simulink model "PV_Battery_MPC"  (R2025a)
settings: Solver=ode4  StartTime=0.0  StopTime=ScenarioStopTime  FixedStep=1e-5  RelTol=1e-3
undefined symbols (not defined in the file): ARIMA_Phi_G, ARIMA_Phi_R, ARIMA_Phi_T, BAT_OCV_TABLE, BAT_SOC_BP, ControllerSelect, DC_PI_Ki, DC_PI_Kp, MPC_OV_weights_curtail, MPC_OV_weights_normal, MPPT_P_deadband, MPPT_P_init, MPPT_V_init, MPPT_V_max, MPPT_V_min, MPPT_V_step, OperatingPointInfo, PV_G_BP, PV_I_TABLE, PV_PI_Ki, PV_PI_Kp, PV_T_BP, PV_V_BP, PVBATT_P, u0, w0, x0
libraries: mpclib x1
settings Model: Creator=Limingyu  LastModifiedBy=Limingyu
settings DataIOCC: SaveOutput=off  SignalLogging=off

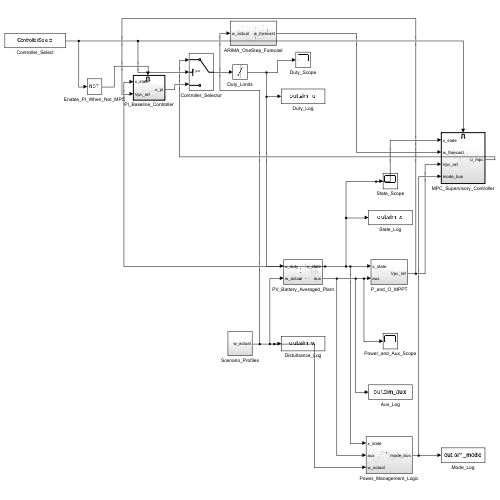
[thumbnail: Simulink's stored preview of the top-level diagram]
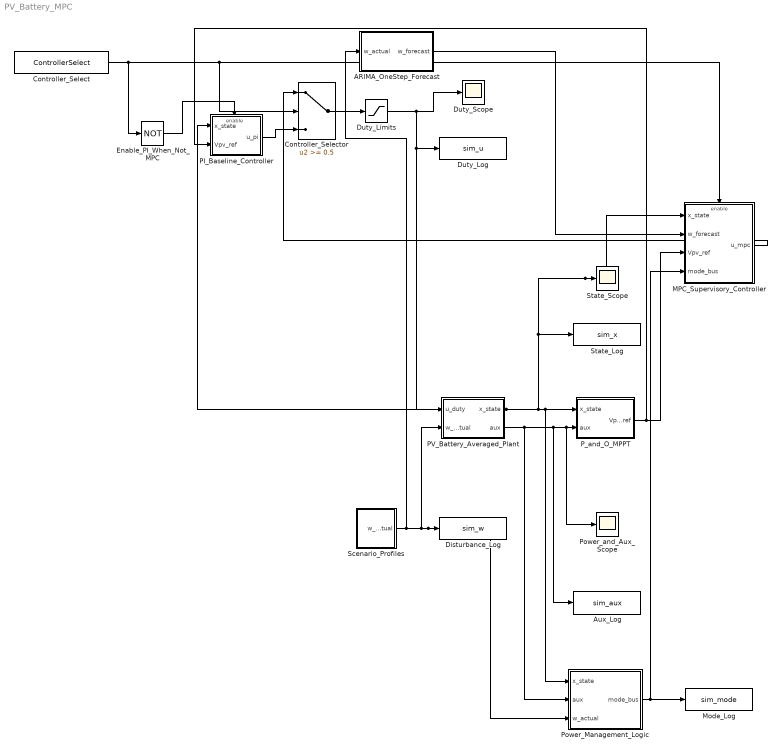
== system PV_Battery_MPC ==
  ARIMA_OneStep_Forecast : Subsystem
  Aux_Log : ToWorkspace  VariableName=sim_aux  SaveFormat=Structure With Time
      settings: Decimation=100
  Controller_Select : Constant  Value=ControllerSelect
  Controller_Selector : Switch  Threshold=0.5
  Disturbance_Log : ToWorkspace  VariableName=sim_w  SaveFormat=Structure With Time
      settings: Decimation=100
  Duty_Limits : Saturate  UpperLimit=0.95  LowerLimit=0.02
  Duty_Log : ToWorkspace  VariableName=sim_u  SaveFormat=Structure With Time
      settings: Decimation=100
  Duty_Scope : Scope
  Enable_PI_When_Not_MPC : Logic  Operator=NOT  Inputs=1  AllPortsSameDT=off  OutDataTypeStr=boolean
  MPC_Supervisory_Controller : Subsystem
  Mode_Log : ToWorkspace  VariableName=sim_mode  SaveFormat=Structure With Time
      settings: Decimation=100
  PI_Baseline_Controller : Subsystem
  PV_Battery_Averaged_Plant : Subsystem
  P_and_O_MPPT : Subsystem
  Power_Management_Logic : Subsystem
  Power_and_Aux_Scope : Scope
  Scenario_Profiles : Subsystem
  State_Log : ToWorkspace  VariableName=sim_x  SaveFormat=Structure With Time
      settings: Decimation=100
  State_Scope : Scope
  wires:
  Duty_Limits/1 -> PV_Battery_Averaged_Plant/1(u_duty), Duty_Log/1, Duty_Scope/1
  Controller_Selector/1 -> Duty_Limits/1
  PI_Baseline_Controller/1(u_pi) -> Controller_Selector/3
  Controller_Select/1 -> Controller_Selector/2, MPC_Supervisory_Controller/Enable, Enable_PI_When_Not_MPC/1
  MPC_Supervisory_Controller/1(u_mpc) -> Controller_Selector/1
  Power_Management_Logic/1(mode_bus) -> MPC_Supervisory_Controller/4(mode_bus), Mode_Log/1
  P_and_O_MPPT/1(Vpv_ref) -> PI_Baseline_Controller/2(Vpv_ref), MPC_Supervisory_Controller/3(Vpv_ref)
  ARIMA_OneStep_Forecast/1(w_forecast) -> MPC_Supervisory_Controller/2(w_forecast)
  PV_Battery_Averaged_Plant/2(aux) -> Aux_Log/1, Power_and_Aux_Scope/1, P_and_O_MPPT/2(aux), Power_Management_Logic/2(aux)
  PV_Battery_Averaged_Plant/1(x_state) -> Power_Management_Logic/1(x_state), P_and_O_MPPT/1(x_state), State_Scope/1, MPC_Supervisory_Controller/1(x_state), State_Log/1, PI_Baseline_Controller/1(x_state)
  Scenario_Profiles/1(w_actual) -> PV_Battery_Averaged_Plant/2(w_actual), Disturbance_Log/1, Power_Management_Logic/3(w_actual), ARIMA_OneStep_Forecast/1(w_actual)
  Enable_PI_When_Not_MPC/1 -> PI_Baseline_Controller/Enable

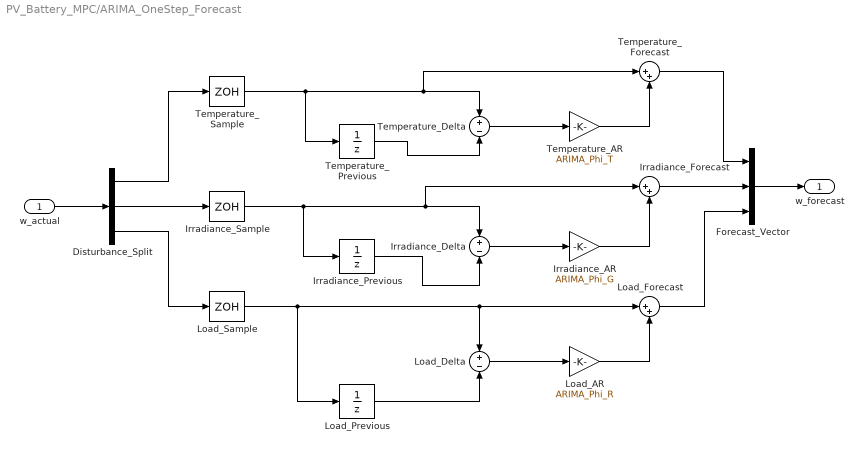
== system PV_Battery_MPC/ARIMA_OneStep_Forecast ==
  w_actual : Inport
  Disturbance_Split : Demux  Outputs=3
  Forecast_Vector : Mux  Inputs=3
  Irradiance_AR : Gain  Gain=ARIMA_Phi_G
  Irradiance_Delta : Sum  Inputs=+-
  Irradiance_Forecast : Sum  Inputs=|++
  Irradiance_Previous : UnitDelay  InitialCondition=w0(2)  SampleTime=0.01
  Irradiance_Sample : ZeroOrderHold  SampleTime=0.01
  Load_AR : Gain  Gain=ARIMA_Phi_R
  Load_Delta : Sum  Inputs=+-
  Load_Forecast : Sum  Inputs=|++
  Load_Previous : UnitDelay  InitialCondition=w0(3)  SampleTime=0.01
  Load_Sample : ZeroOrderHold  SampleTime=0.01
  Temperature_AR : Gain  Gain=ARIMA_Phi_T
  Temperature_Delta : Sum  Inputs=+-
  Temperature_Forecast : Sum  Inputs=|++
  Temperature_Previous : UnitDelay  InitialCondition=w0(1)  SampleTime=0.01
  Temperature_Sample : ZeroOrderHold  SampleTime=0.01
  w_forecast : Outport
  wires:
  Forecast_Vector/1 -> w_forecast/1
  Load_Forecast/1 -> Forecast_Vector/3
  Irradiance_Forecast/1 -> Forecast_Vector/2
  Temperature_Forecast/1 -> Forecast_Vector/1
  Load_AR/1 -> Load_Forecast/2
  Load_Delta/1 -> Load_AR/1
  Load_Previous/1 -> Load_Delta/2
  Load_Sample/1 -> Load_Delta/1, Load_Forecast/1, Load_Previous/1
  Disturbance_Split/3 -> Load_Sample/1
  Irradiance_AR/1 -> Irradiance_Forecast/2
  Irradiance_Delta/1 -> Irradiance_AR/1
  Irradiance_Previous/1 -> Irradiance_Delta/2
  Irradiance_Sample/1 -> Irradiance_Delta/1, Irradiance_Forecast/1, Irradiance_Previous/1
  Disturbance_Split/2 -> Irradiance_Sample/1
  Temperature_AR/1 -> Temperature_Forecast/2
  Temperature_Delta/1 -> Temperature_AR/1
  Temperature_Previous/1 -> Temperature_Delta/2
  Temperature_Sample/1 -> Temperature_Delta/1, Temperature_Forecast/1, Temperature_Previous/1
  Disturbance_Split/1 -> Temperature_Sample/1
  w_actual/1 -> Disturbance_Split/1

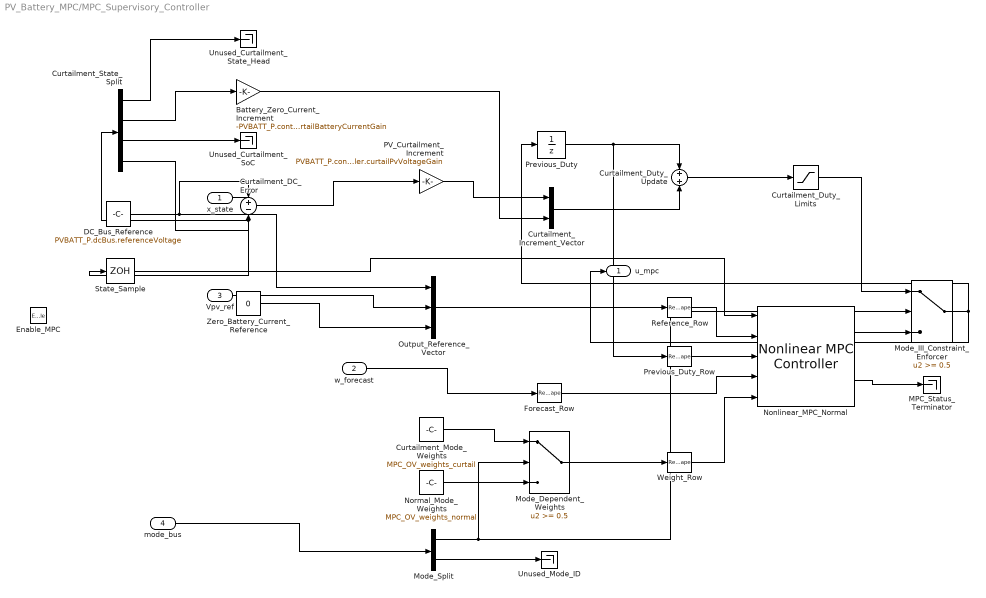
== system PV_Battery_MPC/MPC_Supervisory_Controller ==
  x_state : Inport
  w_forecast : Inport  Port=2
  Vpv_ref : Inport  Port=3
  mode_bus : Inport  Port=4
  Enable_MPC : EnablePort
  Battery_Zero_Current_Increment : Gain  Gain=-PVBATT_P.controller.curtailBatteryCurrentGain
  Curtailment_DC_Error : Sum  Inputs=+-
  Curtailment_Duty_Limits : Saturate  UpperLimit=0.95  LowerLimit=0.02
  Curtailment_Duty_Update : Sum
  Curtailment_Increment_Vector : Mux  Inputs=2
  Curtailment_Mode_Weights : Constant  Value=MPC_OV_weights_curtail
  Curtailment_State_Split : Demux  Outputs=[3 1 1 1]
  DC_Bus_Reference : Constant  Value=PVBATT_P.dcBus.referenceVoltage
  Forecast_Row : Reshape  OutputDimensionality=Customize  OutputDimensions=[1 3]
  MPC_Status_Terminator : Terminator
  Mode_Dependent_Weights : Switch  Threshold=0.5
  Mode_III_Constraint_Enforcer : Switch  Threshold=0.5
  Mode_Split : Demux  Outputs=2
  Nonlinear_MPC_Normal : mpclib/Nonlinear MPC Controller  nlmpcobj=nlmpcobj_pvbatt  UseObjectTs=on  UseMEX=off  md_enabled=on  mvtarget_enabled=off  param_enabled=off  cost_enabled=off  mvseq_enabled=off  stateseq_enabled=off  ovseq_enabled=off  slack_enabled=off  status_enabled=on  ov_min=off  ov_max=off  mv_min=off  mv_max=off  mvrate_min=off  mvrate_max=off  state_min=off  state_max=off  ov_weight=on  mv_weight=off  mvrate_weight=off  ecr_weight=off  nlp_initialize=off
  Normal_Mode_Weights : Constant  Value=MPC_OV_weights_normal
  Output_Reference_Vector : Mux  Inputs=3
  PV_Curtailment_Increment : Gain  Gain=PVBATT_P.controller.curtailPvVoltageGain
  Previous_Duty : UnitDelay  InitialCondition=u0  SampleTime=0.01
  Previous_Duty_Row : Reshape  OutputDimensionality=Customize  OutputDimensions=[1 2]
  Reference_Row : Reshape  OutputDimensionality=Customize  OutputDimensions=[1 3]
  State_Sample : ZeroOrderHold  SampleTime=0.01
  Unused_Curtailment_SoC : Terminator
  Unused_Curtailment_State_Head : Terminator
  Unused_Mode_ID : Terminator
  Weight_Row : Reshape  OutputDimensionality=Customize  OutputDimensions=[1 3]
  Zero_Battery_Current_Reference : Constant  Value=0
  u_mpc : Outport
  wires:
  Nonlinear_MPC_Normal/2 -> MPC_Status_Terminator/1
  Normal_Mode_Weights/1 -> Mode_Dependent_Weights/3
  Mode_Split/1 -> Mode_III_Constraint_Enforcer/2, Mode_Dependent_Weights/2
  Curtailment_Mode_Weights/1 -> Mode_Dependent_Weights/1
  Mode_Split/2 -> Unused_Mode_ID/1
  mode_bus/1 -> Mode_Split/1
  Zero_Battery_Current_Reference/1 -> Output_Reference_Vector/3
  Vpv_ref/1 -> Output_Reference_Vector/2
  DC_Bus_Reference/1 -> Output_Reference_Vector/1, Curtailment_DC_Error/1
  State_Sample/1 -> Nonlinear_MPC_Normal/1
  x_state/1 -> State_Sample/1, Curtailment_State_Split/1
  Output_Reference_Vector/1 -> Reference_Row/1
  Reference_Row/1 -> Nonlinear_MPC_Normal/2
  Previous_Duty/1 -> Curtailment_Duty_Update/1, Previous_Duty_Row/1
  Previous_Duty_Row/1 -> Nonlinear_MPC_Normal/3
  w_forecast/1 -> Forecast_Row/1
  Forecast_Row/1 -> Nonlinear_MPC_Normal/4
  Mode_Dependent_Weights/1 -> Weight_Row/1
  Weight_Row/1 -> Nonlinear_MPC_Normal/5
  Curtailment_State_Split/1 -> Unused_Curtailment_State_Head/1
  Curtailment_State_Split/3 -> Unused_Curtailment_SoC/1
  Curtailment_State_Split/4 -> Curtailment_DC_Error/2
  Curtailment_DC_Error/1 -> PV_Curtailment_Increment/1
  Curtailment_State_Split/2 -> Battery_Zero_Current_Increment/1
  PV_Curtailment_Increment/1 -> Curtailment_Increment_Vector/1
  Battery_Zero_Current_Increment/1 -> Curtailment_Increment_Vector/2
  Curtailment_Increment_Vector/1 -> Curtailment_Duty_Update/2
  Curtailment_Duty_Update/1 -> Curtailment_Duty_Limits/1
  Curtailment_Duty_Limits/1 -> Mode_III_Constraint_Enforcer/1
  Nonlinear_MPC_Normal/1 -> Mode_III_Constraint_Enforcer/3
  Mode_III_Constraint_Enforcer/1 -> u_mpc/1, Previous_Duty/1

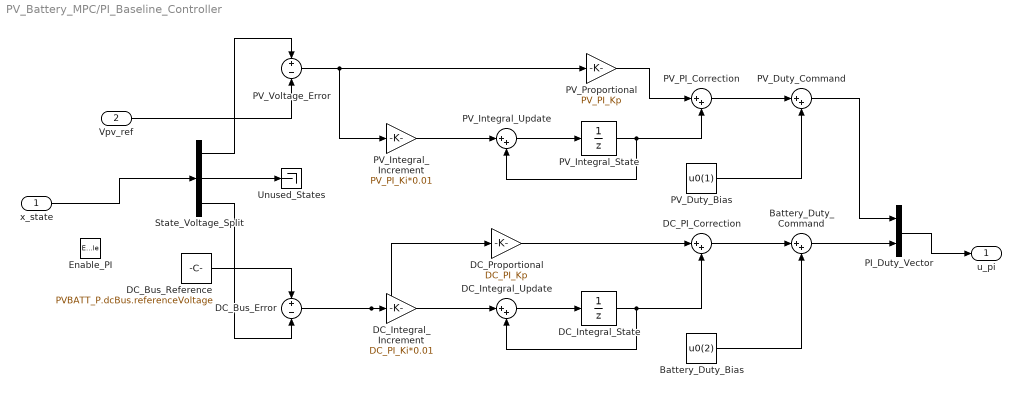
== system PV_Battery_MPC/PI_Baseline_Controller ==
  x_state : Inport
  Vpv_ref : Inport  Port=2
  Enable_PI : EnablePort
  Battery_Duty_Bias : Constant  Value=u0(2)
  Battery_Duty_Command : Sum  Inputs=|++
  DC_Bus_Error : Sum  Inputs=+-
  DC_Bus_Reference : Constant  Value=PVBATT_P.dcBus.referenceVoltage
  DC_Integral_Increment : Gain  Gain=DC_PI_Ki*0.01
  DC_Integral_State : UnitDelay  SampleTime=0.01
  DC_Integral_Update : Sum  Inputs=|++
  DC_PI_Correction : Sum  Inputs=|++
  DC_Proportional : Gain  Gain=DC_PI_Kp
  PI_Duty_Vector : Mux  Inputs=2
  PV_Duty_Bias : Constant  Value=u0(1)
  PV_Duty_Command : Sum  Inputs=|++
  PV_Integral_Increment : Gain  Gain=PV_PI_Ki*0.01
  PV_Integral_State : UnitDelay  SampleTime=0.01
  PV_Integral_Update : Sum  Inputs=|++
  PV_PI_Correction : Sum  Inputs=|++
  PV_Proportional : Gain  Gain=PV_PI_Kp
  PV_Voltage_Error : Sum  Inputs=+-
  State_Voltage_Split : Demux  Outputs=[1 4 1]
  Unused_States : Terminator
  u_pi : Outport
  wires:
  PI_Duty_Vector/1 -> u_pi/1
  Battery_Duty_Command/1 -> PI_Duty_Vector/2
  PV_Duty_Command/1 -> PI_Duty_Vector/1
  Battery_Duty_Bias/1 -> Battery_Duty_Command/2
  DC_PI_Correction/1 -> Battery_Duty_Command/1
  DC_Proportional/1 -> DC_PI_Correction/1
  DC_Integral_Update/1 -> DC_Integral_State/1
  DC_Integral_State/1 -> DC_Integral_Update/2, DC_PI_Correction/2
  DC_Integral_Increment/1 -> DC_Integral_Update/1
  DC_Bus_Error/1 -> DC_Proportional/1, DC_Integral_Increment/1
  State_Voltage_Split/3 -> DC_Bus_Error/2
  DC_Bus_Reference/1 -> DC_Bus_Error/1
  PV_Duty_Bias/1 -> PV_Duty_Command/2
  PV_PI_Correction/1 -> PV_Duty_Command/1
  PV_Proportional/1 -> PV_PI_Correction/1
  PV_Integral_Update/1 -> PV_Integral_State/1
  PV_Integral_State/1 -> PV_Integral_Update/2, PV_PI_Correction/2
  PV_Integral_Increment/1 -> PV_Integral_Update/1
  PV_Voltage_Error/1 -> PV_Integral_Increment/1, PV_Proportional/1
  Vpv_ref/1 -> PV_Voltage_Error/2
  State_Voltage_Split/1 -> PV_Voltage_Error/1
  State_Voltage_Split/2 -> Unused_States/1
  x_state/1 -> State_Voltage_Split/1

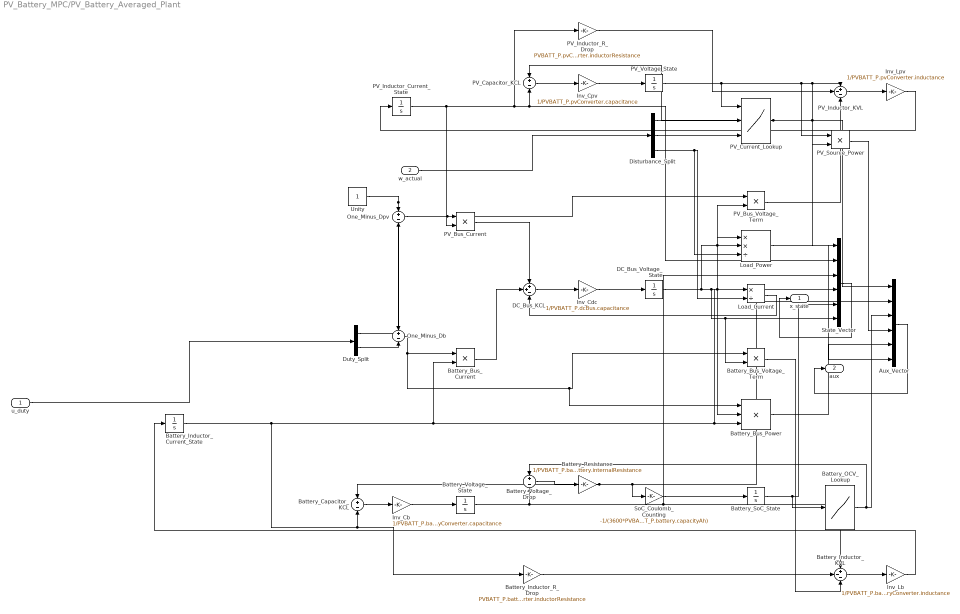
== system PV_Battery_MPC/PV_Battery_Averaged_Plant ==
  u_duty : Inport
  w_actual : Inport  Port=2
  Aux_Vector : Mux  Inputs=6
  Battery_Bus_Current : Product  Inputs=**
  Battery_Bus_Power : Product  Inputs=***
  Battery_Bus_Voltage_Term : Product  Inputs=**
  Battery_Capacitor_KCL : Sum  Inputs=+-
  Battery_Inductor_Current_State : Integrator  InitialCondition=x0(4)
  Battery_Inductor_KVL : Sum  Inputs=+--
  Battery_Inductor_R_Drop : Gain  Gain=PVBATT_P.batteryConverter.inductorResistance
  Battery_OCV_Lookup : Lookup_n-D  NumberOfTableDimensions=1  BreakpointsForDimension1=BAT_SOC_BP  Table=BAT_OCV_TABLE  ExtrapMethod=Clip
  Battery_Resistance : Gain  Gain=1/PVBATT_P.battery.internalResistance
  Battery_SoC_State : Integrator  InitialCondition=x0(5)  LimitOutput=on  UpperSaturationLimit=1  LowerSaturationLimit=0
  Battery_Voltage_Drop : Sum  Inputs=+-
  Battery_Voltage_State : Integrator  InitialCondition=x0(3)
  DC_Bus_KCL : Sum  Inputs=++-
  DC_Bus_Voltage_State : Integrator  InitialCondition=x0(6)
  Disturbance_Split : Demux  Outputs=3
  Duty_Split : Demux  Outputs=2
  Inv_Cb : Gain  Gain=1/PVBATT_P.batteryConverter.capacitance
  Inv_Cdc : Gain  Gain=1/PVBATT_P.dcBus.capacitance
  Inv_Cpv : Gain  Gain=1/PVBATT_P.pvConverter.capacitance
  Inv_Lb : Gain  Gain=1/PVBATT_P.batteryConverter.inductance
  Inv_Lpv : Gain  Gain=1/PVBATT_P.pvConverter.inductance
  Load_Current : Product  Inputs=*/
  Load_Power : Product  Inputs=**/
  One_Minus_Db : Sum  Inputs=+-
  One_Minus_Dpv : Sum  Inputs=+-
  PV_Bus_Current : Product  Inputs=**
  PV_Bus_Voltage_Term : Product  Inputs=**
  PV_Capacitor_KCL : Sum  Inputs=+-
  PV_Current_Lookup : Lookup_n-D  NumberOfTableDimensions=3  BreakpointsForDimension1=PV_V_BP  BreakpointsForDimension2=PV_T_BP  BreakpointsForDimension3=PV_G_BP  Table=PV_I_TABLE  ExtrapMethod=Clip
      settings: InputPortMap=u0,u1,u2
  PV_Inductor_Current_State : Integrator  InitialCondition=x0(2)
  PV_Inductor_KVL : Sum  Inputs=+--
  PV_Inductor_R_Drop : Gain  Gain=PVBATT_P.pvConverter.inductorResistance
  PV_Source_Power : Product  Inputs=**
  PV_Voltage_State : Integrator  InitialCondition=x0(1)
  SoC_Coulomb_Counting : Gain  Gain=-1/(3600*PVBATT_P.battery.capacityAh)
  State_Vector : Mux  Inputs=6
  Unity : Constant
  x_state : Outport
  aux : Outport  Port=2
  wires:
  Aux_Vector/1 -> aux/1
  Load_Power/1 -> Aux_Vector/6
  Battery_Bus_Power/1 -> Aux_Vector/5
  PV_Source_Power/1 -> Aux_Vector/4
  State_Vector/1 -> x_state/1
  Inv_Cdc/1 -> DC_Bus_Voltage_State/1
  DC_Bus_KCL/1 -> Inv_Cdc/1
  Load_Current/1 -> DC_Bus_KCL/3
  Battery_Bus_Current/1 -> DC_Bus_KCL/2
  PV_Bus_Current/1 -> DC_Bus_KCL/1
  Disturbance_Split/3 -> Load_Power/3, Load_Current/2
  SoC_Coulomb_Counting/1 -> Battery_SoC_State/1
  Inv_Lb/1 -> Battery_Inductor_Current_State/1
  Battery_Inductor_KVL/1 -> Inv_Lb/1
  Battery_Bus_Voltage_Term/1 -> Battery_Inductor_KVL/3
  Battery_Inductor_R_Drop/1 -> Battery_Inductor_KVL/2
  One_Minus_Db/1 -> Battery_Bus_Voltage_Term/1, Battery_Bus_Power/1, Battery_Bus_Current/1
  Inv_Cb/1 -> Battery_Voltage_State/1
  Battery_Capacitor_KCL/1 -> Inv_Cb/1
  Battery_Inductor_Current_State/1 -> Battery_Capacitor_KCL/2, Battery_Inductor_R_Drop/1, State_Vector/4, Battery_Bus_Power/3, Battery_Bus_Current/2
  Battery_Resistance/1 -> Aux_Vector/2, SoC_Coulomb_Counting/1, Battery_Capacitor_KCL/1
  Battery_Voltage_Drop/1 -> Battery_Resistance/1
  Battery_Voltage_State/1 -> State_Vector/3, Battery_Inductor_KVL/1, Battery_Voltage_Drop/2
  Battery_OCV_Lookup/1 -> Battery_Voltage_Drop/1, Aux_Vector/3
  Battery_SoC_State/1 -> State_Vector/5, Battery_OCV_Lookup/1
  Inv_Lpv/1 -> PV_Inductor_Current_State/1
  PV_Inductor_KVL/1 -> Inv_Lpv/1
  PV_Bus_Voltage_Term/1 -> PV_Inductor_KVL/3
  PV_Inductor_R_Drop/1 -> PV_Inductor_KVL/2
  DC_Bus_Voltage_State/1 -> PV_Bus_Voltage_Term/2, Battery_Bus_Power/2, Load_Current/1, Battery_Bus_Voltage_Term/2, State_Vector/6, Load_Power/2, Load_Power/1
  One_Minus_Dpv/1 -> PV_Bus_Voltage_Term/1, PV_Bus_Current/1
  Inv_Cpv/1 -> PV_Voltage_State/1
  PV_Capacitor_KCL/1 -> Inv_Cpv/1
  PV_Inductor_Current_State/1 -> PV_Inductor_R_Drop/1, PV_Capacitor_KCL/2, State_Vector/2, PV_Bus_Current/2
  PV_Current_Lookup/1 -> Aux_Vector/1, PV_Source_Power/2, PV_Capacitor_KCL/1
  Disturbance_Split/2 -> PV_Current_Lookup/3
  Disturbance_Split/1 -> PV_Current_Lookup/2
  PV_Voltage_State/1 -> PV_Source_Power/1, PV_Inductor_KVL/1, State_Vector/1, PV_Current_Lookup/1
  Duty_Split/2 -> One_Minus_Db/2
  Duty_Split/1 -> One_Minus_Dpv/2
  Unity/1 -> One_Minus_Dpv/1, One_Minus_Db/1
  w_actual/1 -> Disturbance_Split/1
  u_duty/1 -> Duty_Split/1

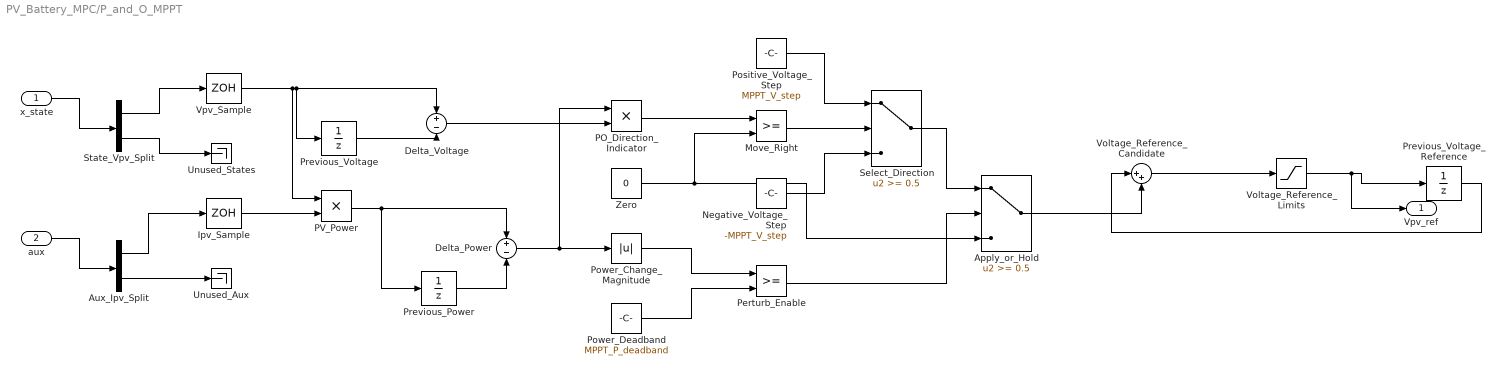
== system PV_Battery_MPC/P_and_O_MPPT ==
  x_state : Inport
  aux : Inport  Port=2
  Apply_or_Hold : Switch  Threshold=0.5
  Aux_Ipv_Split : Demux  Outputs=[1 5]
  Delta_Power : Sum  Inputs=+-
  Delta_Voltage : Sum  Inputs=+-
  Ipv_Sample : ZeroOrderHold  SampleTime=0.01
  Move_Right : RelationalOperator
  Negative_Voltage_Step : Constant  Value=-MPPT_V_step
  PO_Direction_Indicator : Product  Inputs=**
  PV_Power : Product  Inputs=**
  Perturb_Enable : RelationalOperator
  Positive_Voltage_Step : Constant  Value=MPPT_V_step
  Power_Change_Magnitude : Abs
  Power_Deadband : Constant  Value=MPPT_P_deadband
  Previous_Power : UnitDelay  InitialCondition=MPPT_P_init  SampleTime=0.01
  Previous_Voltage : UnitDelay  InitialCondition=MPPT_V_init  SampleTime=0.01
  Previous_Voltage_Reference : UnitDelay  InitialCondition=MPPT_V_init  SampleTime=0.01
  Select_Direction : Switch  Threshold=0.5
  State_Vpv_Split : Demux  Outputs=[1 5]
  Unused_Aux : Terminator
  Unused_States : Terminator
  Voltage_Reference_Candidate : Sum  Inputs=|++
  Voltage_Reference_Limits : Saturate  UpperLimit=MPPT_V_max  LowerLimit=MPPT_V_min
  Vpv_Sample : ZeroOrderHold  SampleTime=0.01
  Zero : Constant  Value=0
  Vpv_ref : Outport
  wires:
  Voltage_Reference_Limits/1 -> Previous_Voltage_Reference/1, Vpv_ref/1
  Voltage_Reference_Candidate/1 -> Voltage_Reference_Limits/1
  Apply_or_Hold/1 -> Voltage_Reference_Candidate/2
  Previous_Voltage_Reference/1 -> Voltage_Reference_Candidate/1
  Perturb_Enable/1 -> Apply_or_Hold/2
  Select_Direction/1 -> Apply_or_Hold/1
  Power_Deadband/1 -> Perturb_Enable/2
  Power_Change_Magnitude/1 -> Perturb_Enable/1
  Negative_Voltage_Step/1 -> Select_Direction/3
  Move_Right/1 -> Select_Direction/2
  Positive_Voltage_Step/1 -> Select_Direction/1
  Zero/1 -> Move_Right/2, Apply_or_Hold/3
  PO_Direction_Indicator/1 -> Move_Right/1
  Delta_Voltage/1 -> PO_Direction_Indicator/2
  Delta_Power/1 -> PO_Direction_Indicator/1, Power_Change_Magnitude/1
  Previous_Voltage/1 -> Delta_Voltage/2
  Previous_Power/1 -> Delta_Power/2
  PV_Power/1 -> Previous_Power/1, Delta_Power/1
  Ipv_Sample/1 -> PV_Power/2
  Vpv_Sample/1 -> PV_Power/1, Previous_Voltage/1, Delta_Voltage/1
  Aux_Ipv_Split/1 -> Ipv_Sample/1
  State_Vpv_Split/1 -> Vpv_Sample/1
  Aux_Ipv_Split/2 -> Unused_Aux/1
  aux/1 -> Aux_Ipv_Split/1
  State_Vpv_Split/2 -> Unused_States/1
  x_state/1 -> State_Vpv_Split/1

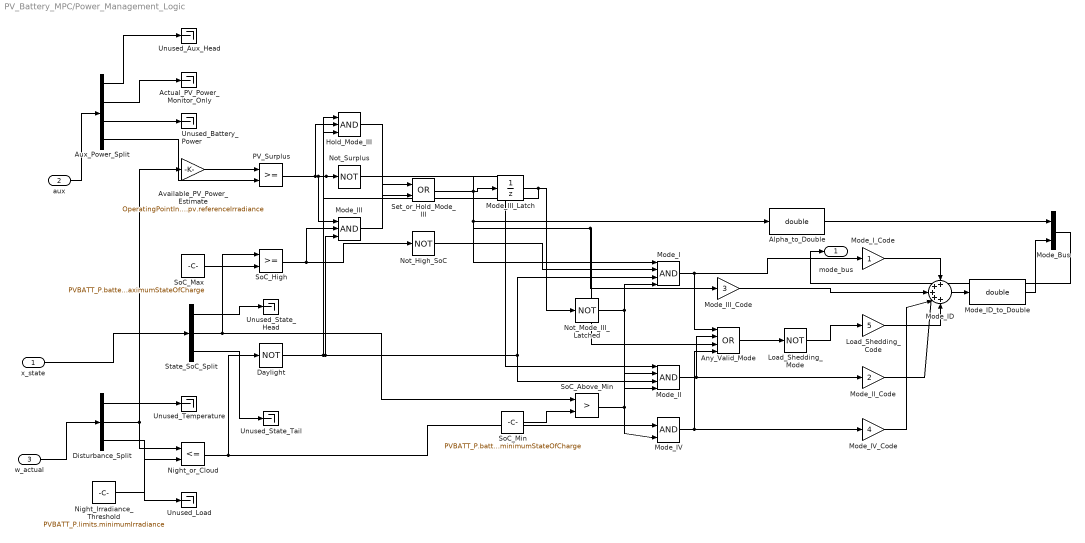
== system PV_Battery_MPC/Power_Management_Logic ==
  x_state : Inport
  aux : Inport  Port=2
  w_actual : Inport  Port=3
  Actual_PV_Power_Monitor_Only : Terminator
  Alpha_to_Double : DataTypeConversion  OutDataTypeStr=double
  Any_Valid_Mode : Logic  Operator=OR  Inputs=4  IconShape=distinctive  AllPortsSameDT=off  OutDataTypeStr=boolean
  Aux_Power_Split : Demux  Outputs=[3 1 1 1]
  Available_PV_Power_Estimate : Gain  Gain=OperatingPointInfo.arrayRatedPower/PVBATT_P.pv.referenceIrradiance
  Daylight : Logic  Operator=NOT  Inputs=1  IconShape=distinctive  AllPortsSameDT=off  OutDataTypeStr=boolean
  Disturbance_Split : Demux  Outputs=3
  Hold_Mode_III : Logic  Inputs=3  AllPortsSameDT=off  OutDataTypeStr=boolean
  Load_Shedding_Code : Gain  Gain=5
  Load_Shedding_Mode : Logic  Operator=NOT  Inputs=1  IconShape=distinctive  AllPortsSameDT=off  OutDataTypeStr=boolean
  Mode_Bus : Mux  Inputs=2
  Mode_I : Logic  Inputs=4  IconShape=distinctive  AllPortsSameDT=off  OutDataTypeStr=boolean
  Mode_ID : Sum  Inputs=+++++
  Mode_ID_to_Double : DataTypeConversion  OutDataTypeStr=double
  Mode_II : Logic  Inputs=4  IconShape=distinctive  AllPortsSameDT=off  OutDataTypeStr=boolean
  Mode_III : Logic  Inputs=3  IconShape=distinctive  AllPortsSameDT=off  OutDataTypeStr=boolean
  Mode_III_Code : Gain  Gain=3
  Mode_III_Latch : UnitDelay  SampleTime=0.01
  Mode_II_Code : Gain  Gain=2
  Mode_IV : Logic  IconShape=distinctive  AllPortsSameDT=off  OutDataTypeStr=boolean
  Mode_IV_Code : Gain  Gain=4
  Mode_I_Code : Gain
  Night_Irradiance_Threshold : Constant  Value=PVBATT_P.limits.minimumIrradiance
  Night_or_Cloud : RelationalOperator  Operator=<=
  Not_High_SoC : Logic  Operator=NOT  Inputs=1  IconShape=distinctive  AllPortsSameDT=off  OutDataTypeStr=boolean
  Not_Mode_III_Latched : Logic  Operator=NOT  Inputs=1  AllPortsSameDT=off  OutDataTypeStr=boolean
  Not_Surplus : Logic  Operator=NOT  Inputs=1  IconShape=distinctive  AllPortsSameDT=off  OutDataTypeStr=boolean
  PV_Surplus : RelationalOperator
  Set_or_Hold_Mode_III : Logic  Operator=OR  AllPortsSameDT=off  OutDataTypeStr=boolean
  SoC_Above_Min : RelationalOperator  Operator=>
  SoC_High : RelationalOperator
  SoC_Max : Constant  Value=PVBATT_P.battery.maximumStateOfCharge
  SoC_Min : Constant  Value=PVBATT_P.battery.minimumStateOfCharge
  State_SoC_Split : Demux  Outputs=[4 1 1]
  Unused_Aux_Head : Terminator
  Unused_Battery_Power : Terminator
  Unused_Load : Terminator
  Unused_State_Head : Terminator
  Unused_State_Tail : Terminator
  Unused_Temperature : Terminator
  mode_bus : Outport
  wires:
  Mode_Bus/1 -> mode_bus/1
  Load_Shedding_Code/1 -> Mode_ID/5
  Mode_IV_Code/1 -> Mode_ID/4
  Mode_III_Code/1 -> Mode_ID/3
  Mode_II_Code/1 -> Mode_ID/2
  Mode_I_Code/1 -> Mode_ID/1
  Load_Shedding_Mode/1 -> Load_Shedding_Code/1
  Any_Valid_Mode/1 -> Load_Shedding_Mode/1
  Mode_IV/1 -> Any_Valid_Mode/4, Mode_IV_Code/1
  Mode_II/1 -> Any_Valid_Mode/2, Mode_II_Code/1
  Mode_I/1 -> Any_Valid_Mode/1, Mode_I_Code/1
  SoC_Above_Min/1 -> Mode_II/2, Mode_IV/2
  Not_Surplus/1 -> Mode_II/1
  Daylight/1 -> Hold_Mode_III/3, Mode_II/3, Mode_I/3, Mode_III/3
  Not_High_SoC/1 -> Mode_I/2
  Night_or_Cloud/1 -> Daylight/1, Mode_IV/1
  SoC_High/1 -> Not_High_SoC/1, Mode_III/2
  PV_Surplus/1 -> Mode_I/1, Not_Surplus/1, Mode_III/1, Hold_Mode_III/2
  Night_Irradiance_Threshold/1 -> Night_or_Cloud/2
  Disturbance_Split/2 -> Available_PV_Power_Estimate/1, Night_or_Cloud/1
  SoC_Min/1 -> SoC_Above_Min/2
  SoC_Max/1 -> SoC_High/2
  State_SoC_Split/2 -> SoC_High/1, SoC_Above_Min/1
  Aux_Power_Split/4 -> PV_Surplus/2
  Disturbance_Split/3 -> Unused_Load/1
  Disturbance_Split/1 -> Unused_Temperature/1
  w_actual/1 -> Disturbance_Split/1
  Aux_Power_Split/3 -> Unused_Battery_Power/1
  Aux_Power_Split/1 -> Unused_Aux_Head/1
  aux/1 -> Aux_Power_Split/1
  State_SoC_Split/3 -> Unused_State_Tail/1
  State_SoC_Split/1 -> Unused_State_Head/1
  x_state/1 -> State_SoC_Split/1
  Alpha_to_Double/1 -> Mode_Bus/1
  Mode_ID/1 -> Mode_ID_to_Double/1
  Mode_ID_to_Double/1 -> Mode_Bus/2
  Available_PV_Power_Estimate/1 -> PV_Surplus/1
  Aux_Power_Split/2 -> Actual_PV_Power_Monitor_Only/1
  Mode_III/1 -> Set_or_Hold_Mode_III/1
  Mode_III_Latch/1 -> Hold_Mode_III/1, Not_Mode_III_Latched/1
  Hold_Mode_III/1 -> Set_or_Hold_Mode_III/2
  Set_or_Hold_Mode_III/1 -> Mode_III_Code/1, Any_Valid_Mode/3, Alpha_to_Double/1, Mode_III_Latch/1
  Not_Mode_III_Latched/1 -> Mode_II/4, Mode_I/4

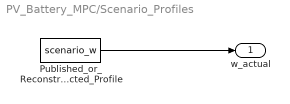
== system PV_Battery_MPC/Scenario_Profiles ==
  Published_or_Reconstructed_Profile : FromWorkspace  VariableName=scenario_w  SampleTime=1e-5  Interpolate=off  OutputAfterFinalValue=Holding final value
  w_actual : Outport
  wires:
  Published_or_Reconstructed_Profile/1 -> w_actual/1
